simulink model "vhf_model_setup"  (R2024a)
settings: Solver=FixedStepAuto  StartTime=0.0  StopTime=9  RelTol=1e-3
PreLoadFcn:
  | run('..\startup.m')
model workspace (MAT data in the model file):
  B = 0.01
  J = 0.1
undefined symbols (not defined in the file): g, M, MAX_MOTOR_POWER, MAX_MOTOR_TORQUE, rpm_grid, rpm_t_grid, targetsMCI, TC_MF_alpha, TC_MF_Kp, TC_MF_N, TC_MF_Td, TC_MF_Ts, throttle_grid, THROTTLE_t, TORQUE, torque_grid
libraries: simulink x2, Solver_SF x1, slpidlib x1
CloseFcn:
  | clear control_info_bus
settings Model: Creator=henri  LastModifiedBy=henri
settings OptimizationCC: ReuseModelBlockBuffer=off
settings DebuggingCC: UnconnectedInputMsg=warning  UnconnectedOutputMsg=warning  UnconnectedLineMsg=warning
settings ModelReferenceCC: EnableRefExpFcnMdlSchedulingChecks=on
settings SFSimCC: SimUserIncludeDirs="\".\\observers\""
settings RTWCC: GPUComputeCapability=3.5  DLArmComputeVersion=19.05

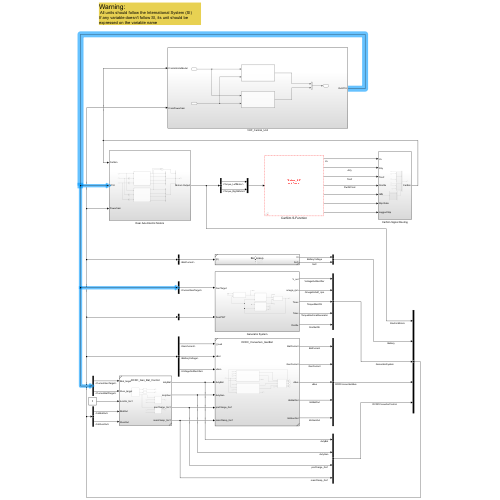
[thumbnail: Simulink's stored preview of the top-level diagram]
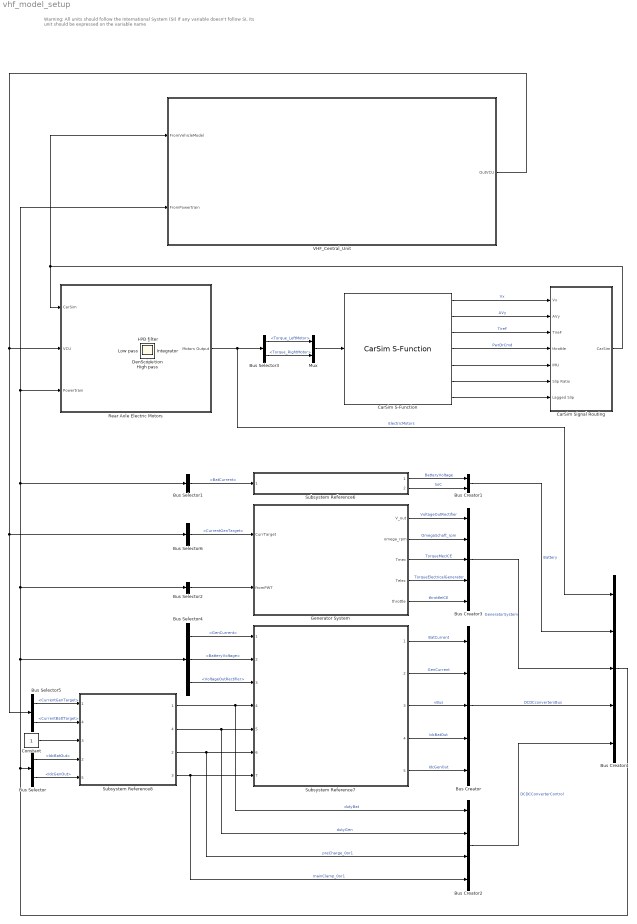
== system vhf_model_setup ==
  note: Warning:
      | All units should follow the International System (SI)
      | If any variable doesn't follow SI, its unit should be expressed on the variable name
  Bus Creator : BusCreator  Inputs=5
  Bus Creator1 : BusCreator  Inputs=2
  Bus Creator2 : BusCreator  Inputs=4
  Bus Creator3 : BusCreator  Inputs=5
  Bus Creator4 : BusCreator  Inputs=5
  Bus Selector : BusSelector  OutputSignals=DCDCconvertersBus.IdcBatOut,DCDCconvertersBus.IdcGenOut
  Bus Selector1 : BusSelector  OutputSignals=DCDCconvertersBus.BatCurrent
  Bus Selector2 : BusSelector  OutputSignals=DCDCconvertersBus.GenCurrent,DCDCconvertersBus.vBus  OutputAsBus=on
  Bus Selector3 : BusSelector  OutputSignals=LeftMotor.Torque_LeftMotor,RightMotor.Torque_RightMotor
  Bus Selector4 : BusSelector  OutputSignals=DCDCconvertersBus.GenCurrent,Battery.BatteryVoltage,GeneratorSystem.VoltageOutRectifier
  Bus Selector5 : BusSelector  OutputSignals=VCU_Powertrain.CurrentGenTarget,VCU_Powertrain.CurrentBattTarget
  Bus Selector6 : BusSelector  OutputSignals=VCU_Powertrain.CurrentGenTarget
  CarSim S-Function : Solver_SF/CarSim S-Function  Priority=1  SIMFILE=simfile.sim  Run_RTs=off  vs_state_ind=Run  StopMode_ind=Vehicle Model
  CarSim Signal Routing : Subsystem
  Constant : Constant
  Generator System : Subsystem
  Mux : Mux  Inputs=2
  Rear Axle Electric Motors : Subsystem
  Subsystem Reference6 : Subsystem  ReferencedSubsystem=Bat_lookup
  Subsystem Reference7 : Subsystem  ReferencedSubsystem=DCDC_Converters_GenBat
  Subsystem Reference8 : Subsystem  ReferencedSubsystem=DCDC_Gen_Bat_Control
      settings: PortSchema="{\"entries\":[{\"content\":{\"sides\":[{\"content\":{\"connectorIds\":[\"In1\",\"In4\",\"In3\",\"In2\",\"In5\"]},\"type\":\"ConnectorPlacement.EquallySpacedRectSide\",\"uuid\":\"07d7d073-649d-4dd5-ba45-9e0b99c3d986\"},{\"content\":{\"connectorIds\":[\"Out1\",\"Out4\",\"Out2\",\"Out3\"],\"side\":\"RIGHT\"},\"type\":\"ConnectorPlacement.EquallySpacedRectSide\",\"uuid\":\"2b65ab9e-6e2c-411c-94b6-50d3edd52af8\"},{\"content\":{\"side\":\"TOP\"},\"type\":\"ConnectorPlacement.EquallySpacedRectSide\",\"uuid\":\"380bd79d-3c3c-4ed9-b669-43271ad9eab7\"}]},\"type\":\"ConnectorPlacement.EquallySpacedConnector\",\"uuid\":\"a384d7c8-4ab4-46be-9278-b103164c1055\"}],\"packageUris\":[\"http://schema.mathworks.com/mf0/Connector/R2020b\"],\"version\":\"1.0\"}"
  VHF_Central_Unit : Subsystem
  Demodulation : Scope
  HPF gain : Scope
  High pass : Scope
  Integrator : Scope
  Low pass : Scope
  PD filter : Scope
  Scope : Scope
  wires:
  Mux/1 -> CarSim S-Function/1
  CarSim S-Function/2 -> CarSim Signal Routing/2(AVy)  "AVy"
  CarSim S-Function/6 -> CarSim Signal Routing/6(Slip Ratio)
  CarSim S-Function/7 -> CarSim Signal Routing/7(Lagged Slip)
  CarSim S-Function/1 -> CarSim Signal Routing/1(Vx)  "Vx"
  CarSim S-Function/3 -> CarSim Signal Routing/3(TireF)  "TireF"
  CarSim S-Function/4 -> CarSim Signal Routing/4(throttle)  "PwrDrCmd"
  CarSim S-Function/5 -> CarSim Signal Routing/5(IMU)
  Subsystem Reference7/1 -> Bus Creator/1  "BatCurrent"
  Subsystem Reference7/2 -> Bus Creator/2  "GenCurrent"
  Subsystem Reference7/3 -> Bus Creator/3  "vBus"
  Subsystem Reference7/4 -> Bus Creator/4  "IdcBatOut"
  Subsystem Reference7/5 -> Bus Creator/5  "IdcGenOut"
  Bus Creator/1 -> Bus Creator4/4  "DCDCconvertersBus"
  Bus Selector/1 -> Subsystem Reference8/2  "<IdcBatOut>"
  Bus Selector/2 -> Subsystem Reference8/5  "<IdcGenOut>"
  Bus Selector1/1 -> Subsystem Reference6/1  "<BatCurrent>"
  Bus Selector2/1 -> Generator System/2(fromPWT)
  CarSim Signal Routing/1(CarSim) -> VHF_Central_Unit/1(FromVehicleModel), Rear Axle Electric Motors/1(CarSim)
  Bus Selector3/1 -> Mux/1  "<Torque_LeftMotor>"
  Bus Selector3/2 -> Mux/2  "<Torque_RightMotor>"
  Subsystem Reference6/1 -> Bus Creator1/1  "BatteryVoltage"
  Subsystem Reference6/2 -> Bus Creator1/2  "SoC"
  Subsystem Reference8/1 -> Bus Creator2/1, Subsystem Reference7/4  "dutyBat"
  Subsystem Reference8/4 -> Bus Creator2/2, Subsystem Reference7/5  "dutyGen"
  Subsystem Reference8/2 -> Bus Creator2/3, Subsystem Reference7/6  "preCharge_0or1"
  Subsystem Reference8/3 -> Bus Creator2/4, Subsystem Reference7/7  "mainClamp_0or1"
  Generator System/5(throttle) -> Bus Creator3/5  "throttleICE"
  Generator System/4(Telec) -> Bus Creator3/4  "TorqueElectricalGenerator"
  Generator System/3(Tmec) -> Bus Creator3/3  "TorqueMecICE"
  Generator System/2(omega_rpm) -> Bus Creator3/2  "OmegaSchaft_rpm"
  Generator System/1(V_out) -> Bus Creator3/1  "VoltageOutRectifier"
  Bus Creator2/1 -> Bus Creator4/5  "DCDCConverterControl"
  Bus Creator3/1 -> Bus Creator4/3  "GeneratorSystem"
  Bus Creator1/1 -> Bus Creator4/2  "Battery"
  Rear Axle Electric Motors/1(Motors Output) -> Bus Selector3/1, Bus Creator4/1  "ElectricMotors"
  Bus Creator4/1 -> VHF_Central_Unit/2(FromPowertrain), Rear Axle Electric Motors/3(Powertrain), Bus Selector1/1, Bus Selector2/1, Bus Selector4/1, Bus Selector/1
  Bus Selector4/1 -> Subsystem Reference7/1  "<GenCurrent>"
  Bus Selector4/2 -> Subsystem Reference7/2  "<BatteryVoltage>"
  Bus Selector4/3 -> Subsystem Reference7/3  "<VoltageOutRectifier>"
  VHF_Central_Unit/1(OutVCU) -> Rear Axle Electric Motors/2(VCU), Bus Selector6/1, Bus Selector5/1
  Bus Selector6/1 -> Generator System/1(CurrTarget)  "<CurrentGenTarget>"
  Bus Selector5/1 -> Subsystem Reference8/1  "<CurrentGenTarget>"
  Bus Selector5/2 -> Subsystem Reference8/4  "<CurrentBattTarget>"
  Constant/1 -> Subsystem Reference8/3

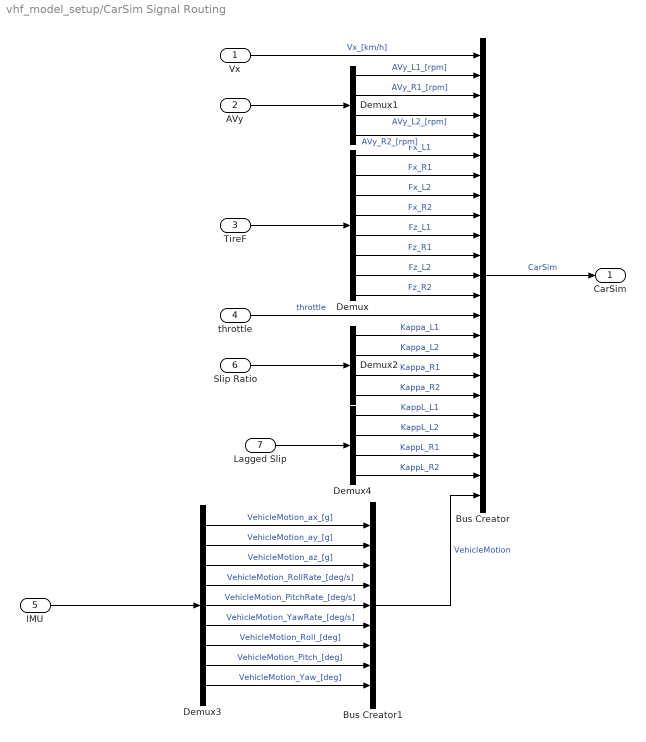
== system vhf_model_setup/CarSim Signal Routing ==
  Vx : Inport
  AVy : Inport  Port=2
  TireF : Inport  Port=3
  throttle : Inport  Port=4
  IMU : Inport  Port=5
  Slip Ratio : Inport  Port=6
  Lagged Slip : Inport  Port=7
  Bus Creator : BusCreator  Inputs=23
  Bus Creator1 : BusCreator  Inputs=9
  Demux : Demux  Outputs=8
  Demux1 : Demux
  Demux2 : Demux
  Demux3 : Demux  Outputs=9
  Demux4 : Demux
  CarSim : Outport
  wires:
  IMU/1 -> Demux3/1
  Bus Creator/1 -> CarSim/1  "CarSim"
  Demux2/4 -> Bus Creator/18  "Kappa_R2"
  Demux2/3 -> Bus Creator/17  "Kappa_R1"
  Slip Ratio/1 -> Demux2/1
  AVy/1 -> Demux1/1
  Demux2/2 -> Bus Creator/16  "Kappa_L2"
  Demux2/1 -> Bus Creator/15  "Kappa_L1"
  Demux/2 -> Bus Creator/7  "Fx_R1"
  Demux1/1 -> Bus Creator/2  "AVy_L1_[rpm]"
  Demux1/2 -> Bus Creator/3  "AVy_R1_[rpm]"
  Demux/1 -> Bus Creator/6  "Fx_L1"
  Demux1/3 -> Bus Creator/4  "AVy_L2_[rpm]"
  TireF/1 -> Demux/1
  Demux1/4 -> Bus Creator/5  "AVy_R2_[rpm]"
  Vx/1 -> Bus Creator/1  "Vx_[km/h]"
  throttle/1 -> Bus Creator/14  "throttle"
  Demux/3 -> Bus Creator/8  "Fx_L2"
  Demux/4 -> Bus Creator/9  "Fx_R2"
  Demux/5 -> Bus Creator/10  "Fz_L1"
  Demux/6 -> Bus Creator/11  "Fz_R1"
  Demux/7 -> Bus Creator/12  "Fz_L2"
  Demux/8 -> Bus Creator/13  "Fz_R2"
  Lagged Slip/1 -> Demux4/1
  Demux4/1 -> Bus Creator/19  "KappL_L1"
  Demux4/2 -> Bus Creator/20  "KappL_L2"
  Demux4/4 -> Bus Creator/22  "KappL_R2"
  Demux4/3 -> Bus Creator/21  "KappL_R1"
  Demux3/1 -> Bus Creator1/1  "VehicleMotion_ax_[g]"
  Demux3/9 -> Bus Creator1/9  "VehicleMotion_Yaw_[deg]"
  Demux3/8 -> Bus Creator1/8  "VehicleMotion_Pitch_[deg]"
  Demux3/7 -> Bus Creator1/7  "VehicleMotion_Roll_[deg]"
  Demux3/6 -> Bus Creator1/6  "VehicleMotion_YawRate_[deg/s]"
  Demux3/5 -> Bus Creator1/5  "VehicleMotion_PitchRate_[deg/s]"
  Demux3/4 -> Bus Creator1/4  "VehicleMotion_RollRate_[deg/s]"
  Demux3/3 -> Bus Creator1/3  "VehicleMotion_az_[g]"
  Demux3/2 -> Bus Creator1/2  "VehicleMotion_ay_[g]"
  Bus Creator1/1 -> Bus Creator/23  "VehicleMotion"

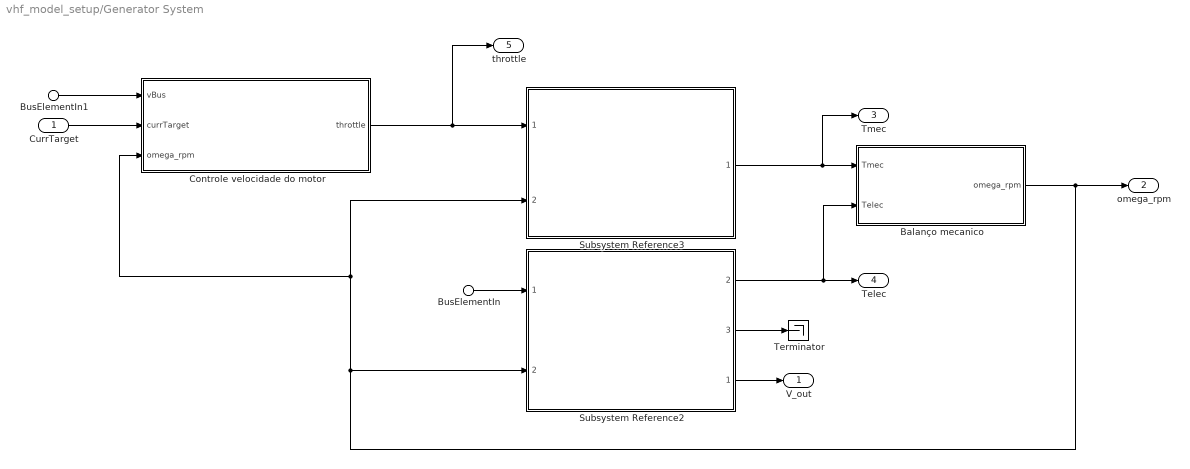
== system vhf_model_setup/Generator System ==
  CurrTarget : Inport
  BusElementIn : Inport  Port=2  PortName=fromPWT  Element=GenCurrent
  BusElementIn1 : Inport  Port=2  PortName=fromPWT  Element=vBus
  Balanço mecanico : Subsystem
  Controle velocidade do motor : Subsystem
  Subsystem Reference2 : Subsystem  ReferencedSubsystem=Generator_V2
      settings: PortSchema="{\"entries\":[{\"content\":{\"sides\":[{\"content\":{\"connectorIds\":[\"In1\",\"In2\"]},\"type\":\"ConnectorPlacement.EquallySpacedRectSide\",\"uuid\":\"e17fb8a6-b9e2-44fc-9782-17160aaa0541\"},{\"content\":{\"connectorIds\":[\"Out2\",\"Out3\",\"Out1\"],\"side\":\"RIGHT\"},\"type\":\"ConnectorPlacement.EquallySpacedRectSide\",\"uuid\":\"f152f6b9-0348-4082-b4a6-2a28004d56aa\"},{\"content\":{\"side\":\"TOP\"},\"type\":\"ConnectorPlacement.EquallySpacedRectSide\",\"uuid\":\"84bd3409-1ffd-4a2d-b774-99b7aec6f8d1\"}]},\"type\":\"ConnectorPlacement.EquallySpacedConnector\",\"uuid\":\"86673931-c8c4-4310-9ac3-5a0ca8838b0d\"}],\"packageUris\":[\"http://schema.mathworks.com/mf0/Connector/R2020b\"],\"version\":\"1.0\"}"
  Subsystem Reference3 : Subsystem  ReferencedSubsystem=ICE_lookup_V2
  Terminator : Terminator
  V_out : Outport
  omega_rpm : Outport  Port=2
  Tmec : Outport  Port=3
  Telec : Outport  Port=4
  throttle : Outport  Port=5
  wires:
  BusElementIn/1 -> Subsystem Reference2/1
  Controle velocidade do motor/1(throttle) -> throttle/1, Subsystem Reference3/1
  Subsystem Reference2/2 -> Balanço mecanico/2(Telec), Telec/1
  Subsystem Reference2/1 -> V_out/1
  Subsystem Reference3/1 -> Tmec/1, Balanço mecanico/1(Tmec)
  Balanço mecanico/1(omega_rpm) -> omega_rpm/1, Subsystem Reference2/2, Subsystem Reference3/2, Controle velocidade do motor/3(omega_rpm)
  CurrTarget/1 -> Controle velocidade do motor/2(currTarget)
  BusElementIn1/1 -> Controle velocidade do motor/1(vBus)
  Subsystem Reference2/3 -> Terminator/1

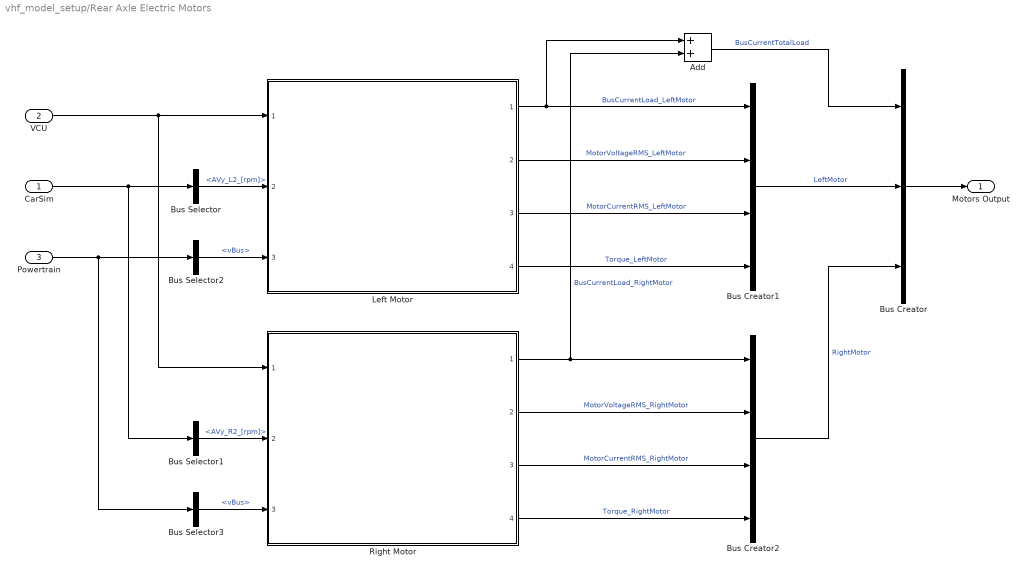
== system vhf_model_setup/Rear Axle Electric Motors ==
  CarSim : Inport
  VCU : Inport  Port=2
  Powertrain : Inport  Port=3
  Add : Sum
  Bus Creator : BusCreator  Inputs=3
  Bus Creator1 : BusCreator  Inputs=4
  Bus Creator2 : BusCreator  Inputs=4
  Bus Selector : BusSelector  OutputSignals=AVy_L2_[rpm]
  Bus Selector1 : BusSelector  OutputSignals=AVy_R2_[rpm]
  Bus Selector2 : BusSelector  OutputSignals=DCDCconvertersBus.vBus
  Bus Selector3 : BusSelector  OutputSignals=DCDCconvertersBus.vBus
  Left Motor : Subsystem  ReferencedSubsystem=Motor
  Right Motor : Subsystem  ReferencedSubsystem=Motor
  Motors Output : Outport
  wires:
  Left Motor/2 -> Bus Creator1/2  "MotorVoltageRMS_LeftMotor"
  VCU/1 -> Right Motor/1, Left Motor/1
  Bus Selector1/1 -> Right Motor/2  "<AVy_R2_[rpm]>"
  Left Motor/1 -> Add/1, Bus Creator1/1  "BusCurrentLoad_LeftMotor"
  CarSim/1 -> Bus Selector/1, Bus Selector1/1
  Bus Selector/1 -> Left Motor/2  "<AVy_L2_[rpm]>"
  Left Motor/3 -> Bus Creator1/3  "MotorCurrentRMS_LeftMotor"
  Left Motor/4 -> Bus Creator1/4  "Torque_LeftMotor"
  Right Motor/1 -> Add/2, Bus Creator2/1  "BusCurrentLoad_RightMotor"
  Right Motor/2 -> Bus Creator2/2  "MotorVoltageRMS_RightMotor"
  Right Motor/3 -> Bus Creator2/3  "MotorCurrentRMS_RightMotor"
  Right Motor/4 -> Bus Creator2/4  "Torque_RightMotor"
  Bus Creator1/1 -> Bus Creator/2  "LeftMotor"
  Bus Creator2/1 -> Bus Creator/3  "RightMotor"
  Add/1 -> Bus Creator/1  "BusCurrentTotalLoad"
  Bus Creator/1 -> Motors Output/1
  Powertrain/1 -> Bus Selector2/1, Bus Selector3/1
  Bus Selector3/1 -> Right Motor/3  "<vBus>"
  Bus Selector2/1 -> Left Motor/3  "<vBus>"

== system vhf_model_setup/VHF_Central_Unit ==
  FromVehicleModel : Inport
  FromPowertrain : Inport  Port=2
  ASW_Chassis : Subsystem  TreatAsAtomicUnit=on
  ASW_Powertrain : Subsystem  TreatAsAtomicUnit=on
  Bus Creator : BusCreator  Inputs=2
  OutVCU : Outport
  wires:
  FromVehicleModel/1 -> ASW_Powertrain/1(SignalInputs), ASW_Chassis/1(SignalInputs)
  ASW_Chassis/1(throttle_motors) -> Bus Creator/1  "VCU_Chassis"
  ASW_Powertrain/1(SignalOutputs) -> Bus Creator/2  "VCU_Powertrain"
  Bus Creator/1 -> OutVCU/1
  FromPowertrain/1 -> ASW_Chassis/2(FromPowertrain), ASW_Powertrain/2(FromPowertrain)

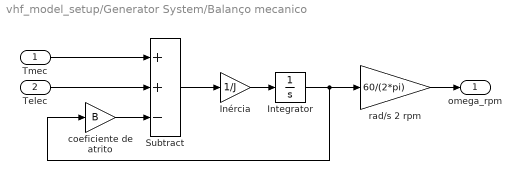
== system vhf_model_setup/Generator System/Balanço mecanico ==
  Tmec : Inport
  Telec : Inport  Port=2
  Integrator : Integrator
  Inércia : Gain  Gain=1/J
  Subtract : Sum  Inputs=++-
  coeficiente de atrito : Gain  Gain=B
  rad/s 2 rpm : Gain  Gain=60/(2*pi)
  omega_rpm : Outport
  wires:
  Integrator/1 -> coeficiente de atrito/1, rad/s 2 rpm/1
  Tmec/1 -> Subtract/1
  Telec/1 -> Subtract/2
  Inércia/1 -> Integrator/1
  Subtract/1 -> Inércia/1
  coeficiente de atrito/1 -> Subtract/3
  rad/s 2 rpm/1 -> omega_rpm/1

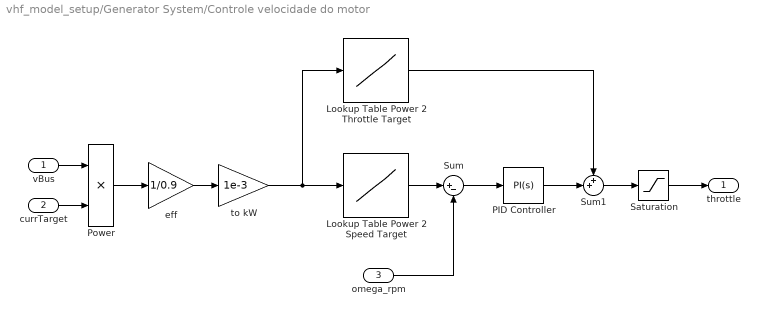
== system vhf_model_setup/Generator System/Controle velocidade do motor ==
  vBus : Inport
  currTarget : Inport  Port=2
  omega_rpm : Inport  Port=3
  " Lookup Table Power 2 Speed Target" : Lookup_n-D  NumberOfTableDimensions=1  BreakpointsForDimension1=targetsMCI.Power  Table=targetsMCI.Speed  InternalRulePriority=Speed  RndMeth=Simplest
  " Lookup Table Power 2 Throttle Target" : Lookup_n-D  NumberOfTableDimensions=1  BreakpointsForDimension1=targetsMCI.Power  Table=targetsMCI.Throttle  InternalRulePriority=Speed  RndMeth=Simplest
  PID Controller : slpidlib/PID Controller  Controller=PI  Form=Parallel  TimeDomain=Continuous-time  UseExternalTs=off  SampleTime=-1  IntegratorMethod=Forward Euler  FilterMethod=Forward Euler  ControllerParametersSource=internal  P=0.1  I=0.2  UseKiTs=off  D=0  UseExternalDerivativeSource=off  N=100  UseFilter=on  TunerSelectOption=Transfer Function Based (PID Tuner App)  InitialConditionSource=internal  InitialConditionForIntegrator=0  InitialConditionForFilter=0  DifferentiatorICPrevScaledInput=0  ExternalReset=none  TrackingMode=off  Kt=1  LimitOutput=on  SatLimitsSource=internal  UpperSaturationLimit=90  LowerSaturationLimit=-90  LinearizeAsGain=on  AntiWindupMode=clamping  Kb=1  LimitIntegrator=on  UpperIntegratorSaturationLimit=90  LowerIntegratorSaturationLimit=-90  POutMin=[]  POutMax=[]  IOutMin=[]  IOutMax=[]  DOutMin=[]  DOutMax=[]  NOutMin=[]  NOutMax=[]  SumOutMin=[]  SumOutMax=[]  SaturationOutMin=[]  SaturationOutMax=[]  PParamMin=[]  PParamMax=[]  IParamMin=[]  IParamMax=[]  DParamMin=[]  DParamMax=[]  NParamMin=[]  NParamMax=[]  KbParamMin=[]  KbParamMax=[]  KtParamMin=[]  KtParamMax=[]  KbOutMin=[]  KbOutMax=[]  KtOutMin=[]  KtOutMax=[]  IntegratorOutMin=[]  IntegratorOutMax=[]  FilterOutMin=[]  FilterOutMax=[]  SumI1OutMin=[]  SumI1OutMax=[]  SumI2OutMin=[]  SumI2OutMax=[]  SumI3OutMin=[]  SumI3OutMax=[]  SumI4OutMin=[]  SumI4OutMax=[]  SumDOutMin=[]  SumDOutMax=[]  DifferentiatorOutMin=[]  DifferentiatorOutMax=[]  FilterDiffOutCoefMin=[]  FilterDiffOutCoefMax=[]  ReciprocalOutMin=[]  ReciprocalOutMax=[]  SumDenOutMin=[]  SumDenOutMax=[]  SumNumOutMin=[]  SumNumOutMax=[]  DivideOutMin=[]  DivideOutMax=[]  UdiffTsProdOutMin=[]  UdiffTsProdOutMax=[]  NTsProdOutMin=[]  NTsProdOutMax=[]  UintegralTsProdOutMin=[]  UintegralTsProdOutMax=[]  UngainTsProdOutMin=[]  UngainTsProdOutMax=[]  ClampingZeroOutDataTypeStr=Inherit: Inherit via back propagation  ClampingZeroOutMin=[]  ClampingZeroOutMax=[]  FilterDenConstantOutDataTypeStr=Inherit: Inherit via back propagation  FilterDenConstantOutMin=[]  FilterDenConstantOutMax=[]  PCopyOutDataTypeStr=Inherit: Inherit via back propagation  PCopyOutMin=[]  PCopyOutMax=[]  NCopyOutDataTypeStr=Inherit: Inherit via back propagation  NCopyOutMin=[]  NCopyOutMax=[]  IntegratorContinuousStateAttributes=''  IntegratorStateMustResolveToSignalObject=off  IntegratorRTWStateStorageClass=Auto  FilterContinuousStateAttributes=''  FilterStateMustResolveToSignalObject=off  FilterRTWStateStorageClass=Auto  ParallelPVariant=InternalParameters  IdealPVariant=Disabled  IVariant=InternalParameters  DVariant=Disabled  IntegratorVariant=Continuous  SatVariant=Enabled  AWVariant=ContClampingParallel  PCopyVariant=Disabled  TRVariant=Disabled  FdbkBlocksVariant=Forward  IdealPFdbkVariant=Disabled  SatFdbkVariant=Disabled  DerivativeFilterVariant=Disabled  NVariant=Disabled  NCopyVariant=Disabled_SignalSpec  FilterICVariant=Disabled  IntegratorICVariant=InternalICs  ExternalResetVariant=Disabled  TRSumVariant=Passthrough  SumFdbkVariant=Disabled  SumVariant=Sum_PI  TsampFilterVariant=InternalTs  TsampNgainVariant=Passthrough  TsampIntegralVariant=Disabled_SignalSpec  ExternalSaturationOutDataTypeStr=Inherit: Same as second input  DerivativeSourceVariant=Disabled
  Power : Product
  Saturation : Saturate  UpperLimit=90  LowerLimit=5
  Sum : Sum  Inputs=|+-
  Sum1 : Sum  Inputs=++|
  eff : Gain  Gain=1/0.9
  to kW : Gain  Gain=1e-3
  throttle : Outport
  wires:
  omega_rpm/1 -> Sum/2
  Sum/1 -> PID Controller/1
  PID Controller/1 -> Sum1/2
  vBus/1 -> Power/1
  currTarget/1 -> Power/2
  Power/1 -> eff/1
  eff/1 -> to kW/1
  " Lookup Table Power 2 Speed Target"/1 -> Sum/1
  Sum1/1 -> Saturation/1
  " Lookup Table Power 2 Throttle Target"/1 -> Sum1/1
  to kW/1 -> " Lookup Table Power 2 Throttle Target"/1, " Lookup Table Power 2 Speed Target"/1
  Saturation/1 -> throttle/1

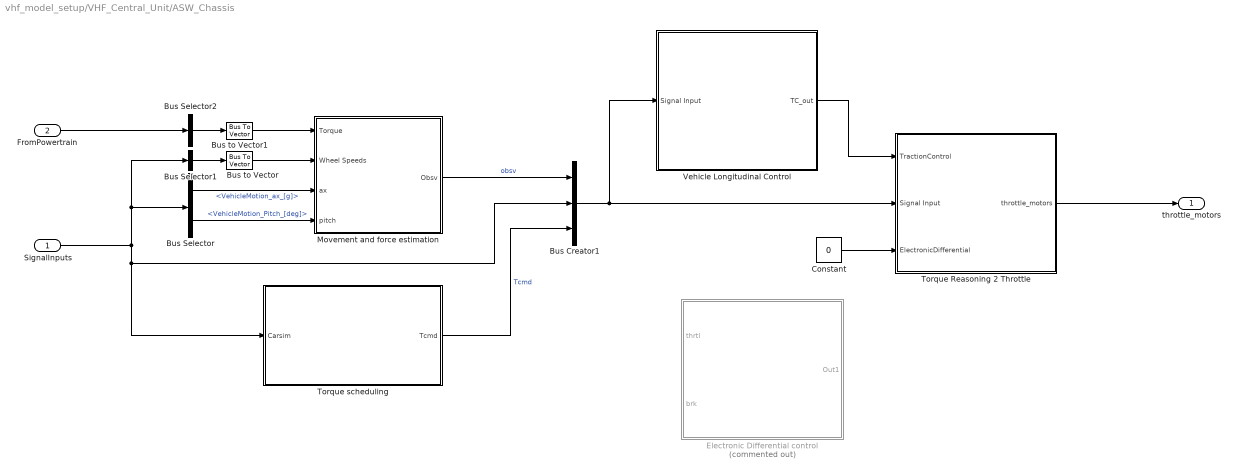
== system vhf_model_setup/VHF_Central_Unit/ASW_Chassis ==
  SignalInputs : Inport
  FromPowertrain : Inport  Port=2
  Bus Creator1 : BusCreator  Inputs=3
  Bus Selector : BusSelector  OutputSignals=VehicleMotion.VehicleMotion_ax_[g],VehicleMotion.VehicleMotion_Pitch_[deg]
  Bus Selector1 : BusSelector  OutputSignals=AVy_L1_[rpm],AVy_R1_[rpm],AVy_L2_[rpm],AVy_R2_[rpm]  OutputAsBus=on
  Bus Selector2 : BusSelector  OutputSignals=ElectricMotors.LeftMotor.Torque_LeftMotor,ElectricMotors.RightMotor.Torque_RightMotor  OutputAsBus=on
  Bus to Vector : BusToVector
  Bus to Vector1 : BusToVector
  Constant : Constant  Value=0
  Electronic Differential control : Subsystem  Commented=on
  Movement and force estimation : Subsystem
  Torque Reasoning 2 Throttle : Subsystem
  Torque scheduling : Subsystem
  Vehicle Longitudinal Control : Subsystem
  throttle_motors : Outport
  wires:
  Bus Creator1/1 -> Vehicle Longitudinal Control/1(Signal Input), Torque Reasoning 2 Throttle/2(Signal Input)
  Movement and force estimation/1(Obsv) -> Bus Creator1/1  "obsv"
  Torque scheduling/1(Tcmd) -> Bus Creator1/3  "Tcmd"
  Bus Selector/1 -> Movement and force estimation/3(ax)  "<VehicleMotion_ax_[g]>"
  Bus Selector/2 -> Movement and force estimation/4(pitch)  "<VehicleMotion_Pitch_[deg]>"
  Bus Selector1/1 -> Bus to Vector/1
  Bus to Vector/1 -> Movement and force estimation/2(Wheel Speeds)
  SignalInputs/1 -> Bus Creator1/2, Torque scheduling/1(Carsim), Bus Selector/1, Bus Selector1/1
  FromPowertrain/1 -> Bus Selector2/1
  Bus Selector2/1 -> Bus to Vector1/1
  Bus to Vector1/1 -> Movement and force estimation/1(Torque)
  Vehicle Longitudinal Control/1(TC_out) -> Torque Reasoning 2 Throttle/1(TractionControl)
  Constant/1 -> Torque Reasoning 2 Throttle/3(ElectronicDifferential)
  Torque Reasoning 2 Throttle/1(throttle_motors) -> throttle_motors/1

== system vhf_model_setup/VHF_Central_Unit/ASW_Powertrain ==
  SignalInputs : Inport
  FromPowertrain : Inport  Port=2
  Bus Creator : BusCreator  Inputs=3
  Bus Selector : BusSelector  OutputSignals=DCDCconvertersBus.vBus,Battery.SoC,ElectricMotors.BusCurrentTotalLoad,GeneratorSystem.VoltageOutRectifier,DCDCconvertersBus.GenCurrent
  Subsystem Reference : Subsystem  ReferencedSubsystem=energy_distribution
      settings: PortSchema="{\"entries\":[{\"content\":{\"sides\":[{\"content\":{\"connectorIds\":[\"In2\",\"In1\",\"In3\",\"In4\",\"In5\"]},\"type\":\"ConnectorPlacement.EquallySpacedRectSide\",\"uuid\":\"5fa4f626-281a-4ff8-baf3-de2b1bbb3a17\"},{\"content\":{\"connectorIds\":[\"Out1\",\"Out2\",\"Out3\"],\"side\":\"RIGHT\"},\"type\":\"ConnectorPlacement.EquallySpacedRectSide\",\"uuid\":\"252f9830-a75c-484b-a352-aea4cbe564ad\"},{\"content\":{\"side\":\"TOP\"},\"type\":\"ConnectorPlacement.EquallySpacedRectSide\",\"uuid\":\"9a86f8a4-ebae-4433-869d-81d154516c9a\"}]},\"type\":\"ConnectorPlacement.EquallySpacedConnector\",\"uuid\":\"0db046dc-65ca-483e-b149-28a932e23f57\"}],\"packageUris\":[\"http://schema.mathworks.com/mf0/Connector/R2020b\"],\"version\":\"1.0\"}"
  Terminator : Terminator
  SignalOutputs : Outport
  wires:
  FromPowertrain/1 -> Bus Selector/1
  Bus Selector/4 -> Subsystem Reference/4  "<VoltageOutRectifier>"
  Bus Selector/3 -> Subsystem Reference/3  "<BusCurrentTotalLoad>"
  Bus Selector/1 -> Subsystem Reference/2  "<vBus>"
  Bus Selector/2 -> Subsystem Reference/1  "<SoC>"
  Bus Selector/5 -> Subsystem Reference/5  "<GenCurrent>"
  SignalInputs/1 -> Terminator/1
  Subsystem Reference/1 -> Bus Creator/1  "CurrentBattTarget"
  Subsystem Reference/2 -> Bus Creator/2  "CurrentLoadTarget"
  Subsystem Reference/3 -> Bus Creator/3  "CurrentGenTarget"
  Bus Creator/1 -> SignalOutputs/1

== system vhf_model_setup/VHF_Central_Unit/ASW_Chassis/Electronic Differential control ==
  thrtl : Inport
  brk : Inport  Port=2
  Constant : Constant
  Terminator : Terminator
  Terminator1 : Terminator
  Out1 : Outport
  wires:
  Constant/1 -> Out1/1
  brk/1 -> Terminator1/1
  thrtl/1 -> Terminator/1

== system vhf_model_setup/VHF_Central_Unit/ASW_Chassis/Movement and force estimation ==
  Torque : Inport
  Wheel Speeds : Inport  Port=2
  ax : Inport  Port=3
  pitch : Inport  Port=4
  Bus Creator : BusCreator  Inputs=3
  Tire forces observer : Subsystem  ReferencedSubsystem=algebraic_PIO_observer
  Obsv : Outport
  wires:
  Bus Creator/1 -> Obsv/1
  pitch/1 -> Tire forces observer/4
  ax/1 -> Tire forces observer/3
  Wheel Speeds/1 -> Tire forces observer/2
  Torque/1 -> Tire forces observer/1
  Tire forces observer/1 -> Bus Creator/1  "wheel_omega_obsv"
  Tire forces observer/2 -> Bus Creator/2  "wheel_Fx_obsv"
  Tire forces observer/3 -> Bus Creator/3  "wheel_Fz_obsv"

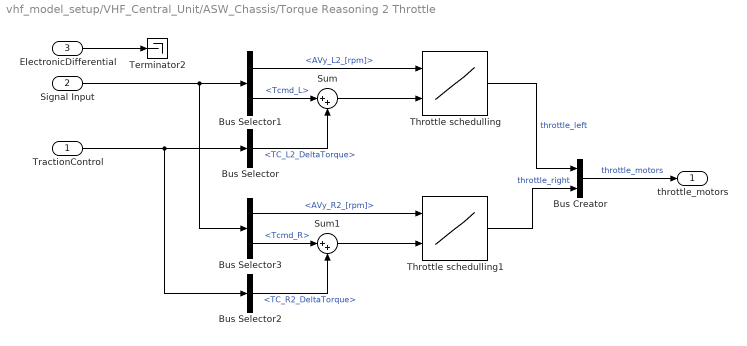
== system vhf_model_setup/VHF_Central_Unit/ASW_Chassis/Torque Reasoning 2 Throttle ==
  TractionControl : Inport
  Signal Input : Inport  Port=2
  ElectronicDifferential : Inport  Port=3
  Bus Creator : BusCreator  Inputs=2
  Bus Selector : BusSelector  OutputSignals=TC_L2_DeltaTorque
  Bus Selector1 : BusSelector  OutputSignals=CarSim.AVy_L2_[rpm],Tcmd.Tcmd_L
  Bus Selector2 : BusSelector  OutputSignals=TC_R2_DeltaTorque
  Bus Selector3 : BusSelector  OutputSignals=CarSim.AVy_R2_[rpm],Tcmd.Tcmd_R
  Sum : Sum  Inputs=|++
  Sum1 : Sum  Inputs=|++
  Terminator2 : Terminator
  Throttle schedulling : Lookup_n-D  BreakpointsForDimension1=rpm_t_grid  BreakpointsForDimension2=torque_grid  BreakpointsForDimension3=[5, 7]  Table=THROTTLE_t  InternalRulePriority=Speed  RndMeth=Simplest
      settings: InputPortMap=u0,u1
  Throttle schedulling1 : Lookup_n-D  BreakpointsForDimension1=rpm_t_grid  BreakpointsForDimension2=torque_grid  BreakpointsForDimension3=[5, 7]  Table=THROTTLE_t  InternalRulePriority=Speed  RndMeth=Simplest
      settings: InputPortMap=u0,u1
  throttle_motors : Outport
  wires:
  Bus Creator/1 -> throttle_motors/1  "throttle_motors"
  Signal Input/1 -> Bus Selector3/1, Bus Selector1/1
  ElectronicDifferential/1 -> Terminator2/1
  TractionControl/1 -> Bus Selector2/1, Bus Selector/1
  Bus Selector1/2 -> Sum/1  "<Tcmd_L>"
  Bus Selector/1 -> Sum/2  "<TC_L2_DeltaTorque>"
  Bus Selector2/1 -> Sum1/2  "<TC_R2_DeltaTorque>"
  Bus Selector3/1 -> Throttle schedulling1/1  "<AVy_R2_[rpm]>"
  Sum/1 -> Throttle schedulling/2
  Bus Selector1/1 -> Throttle schedulling/1  "<AVy_L2_[rpm]>"
  Bus Selector3/2 -> Sum1/1  "<Tcmd_R>"
  Sum1/1 -> Throttle schedulling1/2
  Throttle schedulling/1 -> Bus Creator/1  "throttle_left"
  Throttle schedulling1/1 -> Bus Creator/2  "throttle_right"

== system vhf_model_setup/VHF_Central_Unit/ASW_Chassis/Torque scheduling ==
  Carsim : Inport
  Bus Creator : BusCreator  Inputs=2
  Tcmd Left : Subsystem
  Tcmd Right : Subsystem
  Tcmd : Outport
  wires:
  Bus Creator/1 -> Tcmd/1  "Tcmd"
  Carsim/1 -> Tcmd Right/1(In1), Tcmd Left/1(Carsim)
  Tcmd Left/1(Tcmd_L) -> Bus Creator/1
  Tcmd Right/1(Tcmd_R) -> Bus Creator/2

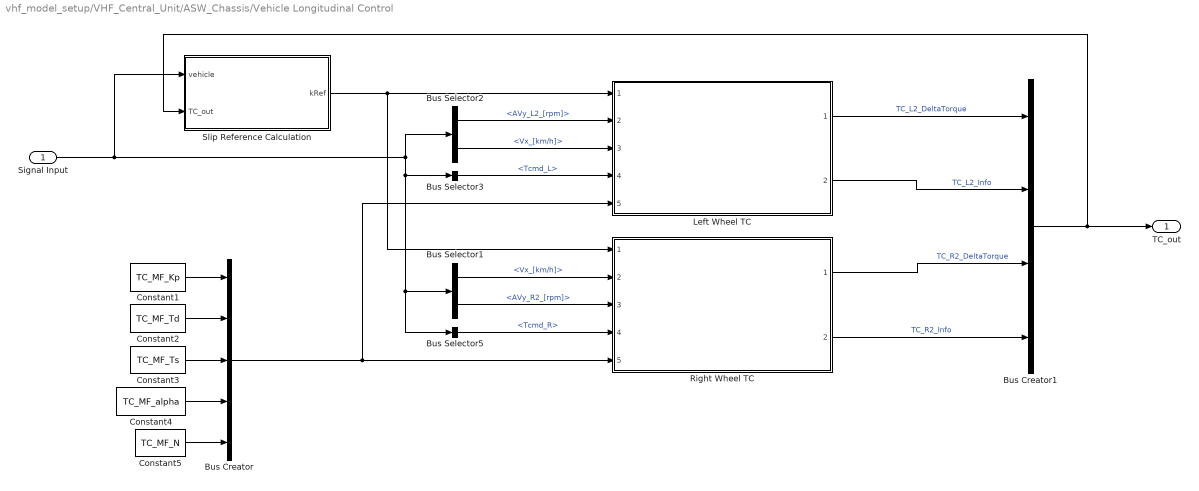
== system vhf_model_setup/VHF_Central_Unit/ASW_Chassis/Vehicle Longitudinal Control ==
  Signal Input : Inport
  Bus Creator : BusCreator  Inputs=5
  Bus Creator1 : BusCreator  Inputs=4
  Bus Selector1 : BusSelector  OutputSignals=CarSim.Vx_[km/h],CarSim.AVy_R2_[rpm]
  Bus Selector2 : BusSelector  OutputSignals=CarSim.AVy_L2_[rpm],CarSim.Vx_[km/h]
  Bus Selector3 : BusSelector  OutputSignals=Tcmd.Tcmd_L
  Bus Selector5 : BusSelector  OutputSignals=Tcmd.Tcmd_R
  Constant1 : Constant  Value=TC_MF_Kp
  Constant2 : Constant  Value=TC_MF_Td
  Constant3 : Constant  Value=TC_MF_Ts
  Constant4 : Constant  Value=TC_MF_alpha
  Constant5 : Constant  Value=TC_MF_N
  Left Wheel TC : Subsystem  ReferencedSubsystem=TractionControlMF
  Right Wheel TC : Subsystem  ReferencedSubsystem=TractionControlMF
  Slip Reference Calculation : Subsystem
  TC_out : Outport
  wires:
  Slip Reference Calculation/1(kRef) -> Left Wheel TC/1, Right Wheel TC/1
  Bus Selector3/1 -> Left Wheel TC/4  "<Tcmd_L>"
  Bus Selector2/1 -> Left Wheel TC/2  "<AVy_L2_[rpm]>"
  Bus Selector2/2 -> Left Wheel TC/3  "<Vx_[km/h]>"
  Bus Selector5/1 -> Right Wheel TC/4  "<Tcmd_R>"
  Bus Selector1/2 -> Right Wheel TC/3  "<AVy_R2_[rpm]>"
  Bus Selector1/1 -> Right Wheel TC/2  "<Vx_[km/h]>"
  Bus Creator/1 -> Right Wheel TC/5, Left Wheel TC/5
  Constant5/1 -> Bus Creator/5
  Constant4/1 -> Bus Creator/4
  Constant3/1 -> Bus Creator/3
  Constant2/1 -> Bus Creator/2
  Constant1/1 -> Bus Creator/1
  Signal Input/1 -> Bus Selector2/1, Bus Selector3/1, Bus Selector1/1, Bus Selector5/1, Slip Reference Calculation/1(vehicle)
  Right Wheel TC/2 -> Bus Creator1/4  "TC_R2_Info"
  Left Wheel TC/1 -> Bus Creator1/1  "TC_L2_DeltaTorque"
  Right Wheel TC/1 -> Bus Creator1/3  "TC_R2_DeltaTorque"
  Left Wheel TC/2 -> Bus Creator1/2  "TC_L2_Info"
  Bus Creator1/1 -> Slip Reference Calculation/2(TC_out), TC_out/1

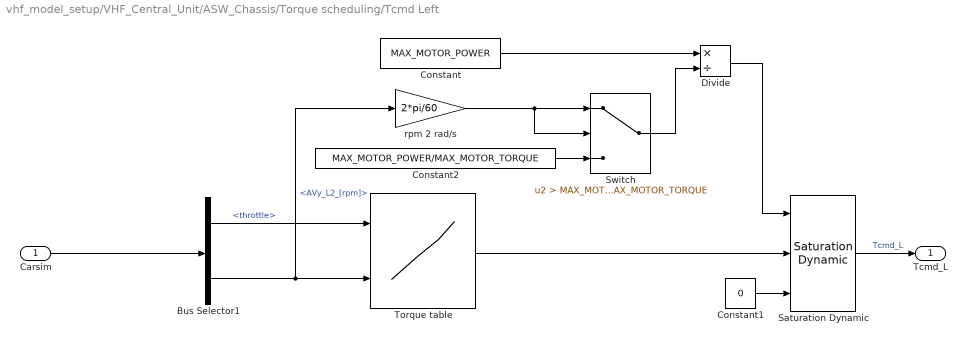
== system vhf_model_setup/VHF_Central_Unit/ASW_Chassis/Torque scheduling/Tcmd Left ==
  Carsim : Inport
  Bus Selector1 : BusSelector  OutputSignals=throttle,AVy_L2_[rpm]
  Constant : Constant  Value=MAX_MOTOR_POWER
  Constant1 : Constant  Value=0
  Constant2 : Constant  Value=MAX_MOTOR_POWER/MAX_MOTOR_TORQUE
  Divide : Product  Inputs=*/
  Saturation Dynamic : simulink/Discontinuities/Saturation Dynamic  OutMin=[]  OutMax=[]  OutDataTypeStr=Inherit: Same as second input  OutDataType=fixdt(1, 16)  OutScaling=2^-10  DoSatur=off
  Switch : Switch  Criteria=u2 > Threshold  Threshold=MAX_MOTOR_POWER/MAX_MOTOR_TORQUE  SaturateOnIntegerOverflow=off  InputSameDT=off
  Torque table : Lookup_n-D  BreakpointsForDimension1=rpm_grid  BreakpointsForDimension2=throttle_grid  Table=TORQUE  InternalRulePriority=Speed  RndMeth=Simplest
      settings: InputPortMap=u0,u1
  rpm 2 rad/s : Gain  Gain=2*pi/60
  Tcmd_L : Outport
  wires:
  Carsim/1 -> Bus Selector1/1
  Constant/1 -> Divide/1
  rpm 2 rad/s/1 -> Switch/2, Switch/1
  Bus Selector1/2 -> rpm 2 rad/s/1, Torque table/2  "<AVy_L2_[rpm]>"
  Constant2/1 -> Switch/3
  Bus Selector1/1 -> Torque table/1  "<throttle>"
  Constant1/1 -> Saturation Dynamic/3
  Switch/1 -> Divide/2
  Divide/1 -> Saturation Dynamic/1
  Saturation Dynamic/1 -> Tcmd_L/1  "Tcmd_L"
  Torque table/1 -> Saturation Dynamic/2

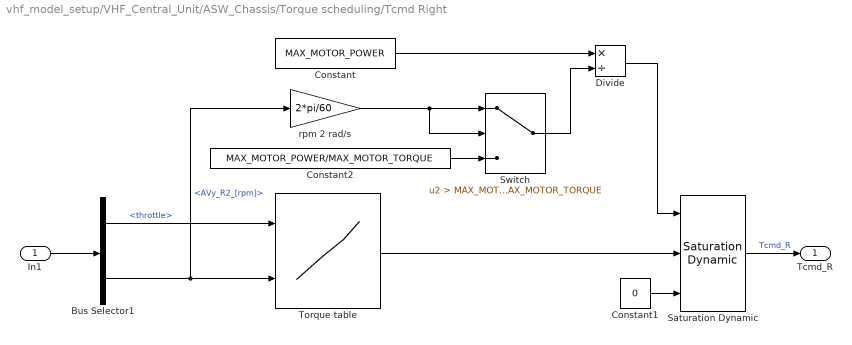
== system vhf_model_setup/VHF_Central_Unit/ASW_Chassis/Torque scheduling/Tcmd Right ==
  In1 : Inport
  Bus Selector1 : BusSelector  OutputSignals=throttle,AVy_R2_[rpm]
  Constant : Constant  Value=MAX_MOTOR_POWER
  Constant1 : Constant  Value=0
  Constant2 : Constant  Value=MAX_MOTOR_POWER/MAX_MOTOR_TORQUE
  Divide : Product  Inputs=*/
  Saturation Dynamic : simulink/Discontinuities/Saturation Dynamic  OutMin=[]  OutMax=[]  OutDataTypeStr=Inherit: Same as second input  OutDataType=fixdt(1, 16)  OutScaling=2^-10  DoSatur=off
  Switch : Switch  Criteria=u2 > Threshold  Threshold=MAX_MOTOR_POWER/MAX_MOTOR_TORQUE  SaturateOnIntegerOverflow=off  InputSameDT=off
  Torque table : Lookup_n-D  BreakpointsForDimension1=rpm_grid  BreakpointsForDimension2=throttle_grid  Table=TORQUE  InternalRulePriority=Speed  RndMeth=Simplest
      settings: InputPortMap=u0,u1
  rpm 2 rad/s : Gain  Gain=2*pi/60
  Tcmd_R : Outport
  wires:
  Saturation Dynamic/1 -> Tcmd_R/1  "Tcmd_R"
  Constant/1 -> Divide/1
  Switch/1 -> Divide/2
  Bus Selector1/1 -> Torque table/1  "<throttle>"
  Bus Selector1/2 -> rpm 2 rad/s/1, Torque table/2  "<AVy_R2_[rpm]>"
  Divide/1 -> Saturation Dynamic/1
  Constant1/1 -> Saturation Dynamic/3
  rpm 2 rad/s/1 -> Switch/2, Switch/1
  Constant2/1 -> Switch/3
  Torque table/1 -> Saturation Dynamic/2
  In1/1 -> Bus Selector1/1

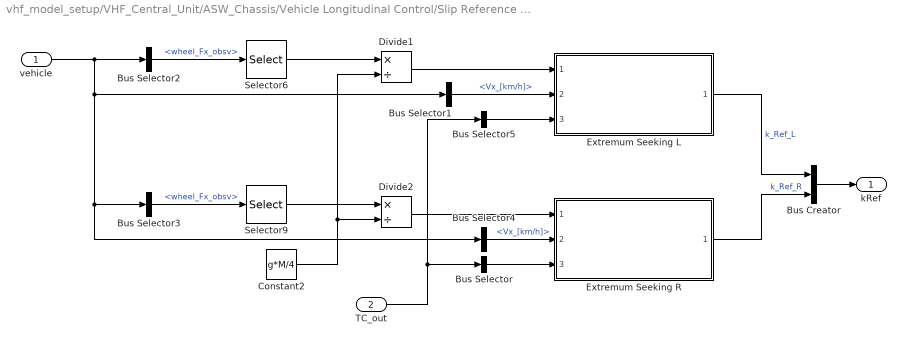
== system vhf_model_setup/VHF_Central_Unit/ASW_Chassis/Vehicle Longitudinal Control/Slip Reference Calculation ==
  vehicle : Inport
  TC_out : Inport  Port=2
  Bus Creator : BusCreator  Inputs=2
  Bus Selector : BusSelector  OutputSignals=TC_R2_Info,TC_L2_Info  OutputAsBus=on
  Bus Selector1 : BusSelector  OutputSignals=CarSim.Vx_[km/h]
  Bus Selector2 : BusSelector  OutputSignals=obsv.wheel_Fx_obsv
  Bus Selector3 : BusSelector  OutputSignals=obsv.wheel_Fx_obsv
  Bus Selector4 : BusSelector  OutputSignals=CarSim.Vx_[km/h]
  Bus Selector5 : BusSelector  OutputSignals=TC_L2_Info,TC_R2_Info  OutputAsBus=on
  Constant2 : Constant  Value=g*M/4
  Divide1 : Product  Inputs=*/
  Divide2 : Product  Inputs=*/
  Extremum Seeking L : Subsystem  ReferencedSubsystem=Extremum_Seeking_vx_gain
  Extremum Seeking R : Subsystem  ReferencedSubsystem=Extremum_Seeking_vx_gain
  Selector6 : Selector  InputPortWidth=4  IndexOptions=Index vector (dialog)  Indices=[3]  OutputSizes=1
  Selector9 : Selector  InputPortWidth=4  IndexOptions=Index vector (dialog)  Indices=[4]  OutputSizes=1
  kRef : Outport
  wires:
  Bus Creator/1 -> kRef/1
  Extremum Seeking R/1 -> Bus Creator/2  "k_Ref_R"
  Divide2/1 -> Extremum Seeking R/1
  Bus Selector3/1 -> Selector9/1  "<wheel_Fx_obsv>"
  Bus Selector2/1 -> Selector6/1  "<wheel_Fx_obsv>"
  vehicle/1 -> Bus Selector1/1, Bus Selector4/1, Bus Selector3/1, Bus Selector2/1
  Selector9/1 -> Divide2/1
  Constant2/1 -> Divide1/2, Divide2/2
  Selector6/1 -> Divide1/1
  Divide1/1 -> Extremum Seeking L/1
  Extremum Seeking L/1 -> Bus Creator/1  "k_Ref_L"
  Bus Selector1/1 -> Extremum Seeking L/2  "<Vx_[km/h]>"
  Bus Selector4/1 -> Extremum Seeking R/2  "<Vx_[km/h]>"
  TC_out/1 -> Bus Selector5/1, Bus Selector/1
  Bus Selector/1 -> Extremum Seeking R/3
  Bus Selector5/1 -> Extremum Seeking L/3
